simulink model "simscape_robot_delta_v8"  (R2024b)
settings: Solver=ode15s  StartTime=0.0  StopTime=20.0  FixedStep=1e-3  RelTol=1e-3
model workspace (MAT data in the model file):
  kd1 = 14
  kd2 = 13.6
  kd3 = 37.9
  ki1 = 39
  ki2 = 36
  ki3 = 11.6
  kp1 = 12.6
  kp2 = 12.2
  kp3 = 14.4
values from neighbouring files (symbols this model uses):
  N = floor(size(err,1)/window)    [grafica_error.m]
undefined symbols (not defined in the file or in its folder): X, Y, Z
libraries: sm_lib x72, nesl_utility x7
(part 3 of 3)

== matlab function simscape_robot_delta_v8/Inverse Kinematics ==
  data: Pd input; phi_d output
function phi_d = CI(Pd)
%%%%%%%%%%%%%%%%%%%%%%%%%%
    Xp=Pd(1);
    Yp=Pd(2);
    Zp=Pd(3);
    %%%%%%%%%%%%%%%%%%%%%%%%%%
    % constantes
    L1 = 0.17;
    L2 = 0.32513;
    ra = 0.1;
    rb = 0.0501;
    r = ra - rb;
    theta = [0; 2*pi/3; -2*pi/3]; 

    E = 2*L1*(r - Xp*cos(theta) - Yp*sin(theta));
    F = -2*L1*Zp*[1;1;1];
    G = Xp^2 + Yp^2 + Zp^2 + r^2 + L1^2 - L2^2 - 2*r*(Xp*cos(theta) + Yp*sin(theta));
    sqrt_val = E.^2 + F.^2 - G.^2;
    phi_d = 2*atan((-F - sqrt(sqrt_val))./( G - E));
end

== matlab function simscape_robot_delta_v8/Direct Kinematics ==
  data: phi input; P output
function P=CD(phi)
     % Constantes 
    L1 = 0.17;
    L2 = 0.32513;
    ra = 0.1;
    rb = 0.0501;
    r = ra - rb;
    theta = [0; 2*pi/3; -2*pi/3]; 

    % Posiciones de las articulaciones pasivas
    X=(r+L1*cos(phi)).*cos(theta);
    Y=(r+L1*cos(phi)).*sin(theta);
    Z=L1*sin(phi);

    if abs(Z(3)-Z(1))<1e-4 && abs(Z(2)-Z(1))<1e-4
        
        % Definimos matriz del sistema de ecuaciones
        M=[2*(X(3)-X(1)),2*(Y(3)-Y(1));
           2*(X(2)-X(1)),2*(Y(2)-Y(1))];
        b=[X(3)^2+Y(3)^2-(X(1)^2+Y(1)^2);
           X(2)^2+Y(2)^2-(X(1)^2+Y(1)^2)];
        w=M\b;
        Xc=w(1);
        Yc=w(2);
        % Calculamos Z
        Zc=Z(1)+sqrt(L2^2-(Xc-X(1))^2-(Yc-Y(1))^2);
        % Guardamos la solución
        P=[Xc;Yc;Zc];

    elseif abs(X(2)-X(3))<1e-5 && abs(Z(3)-Z(2))<1e-5 && abs(X(3)-X(1))>1e-5 && abs(Z(3)-Z(1))>1e-5

        a=-(Z(3)-Z(1))/(X(3)-X(1)); b=(X(3)^2-X(1)^2+Y(3)^2-Y(1)^2+Z(3)^2-Z(1)^2)/(2*(X(3)-X(1)));
        A=a^2+1; B=2*a*(b-X(3))-2*Z(3); C=(b-X(3))^2+Y(3)^2-L2^2+Z(3)^2;
        Zmas=(-B+sqrt(B^2-4*A*C))/(2*A);
        Xmas=a*Zmas+b;
        Ymas=0;
        P=[Xmas;Ymas;Zmas];
        
    else
        % Definimos coeficientes auxiliares
        a11=2*(X(3)-X(1)); a21=2*(X(3)-X(2));
        a12=2*(Y(3)-Y(1)); a22=2*(Y(3)-Y(2));
        a13=2*(Z(3)-Z(1)); a23=2*(Z(3)-Z(2));

        b1=X(3)^2+Y(3)^2+Z(3)^2-(X(1)^2+Y(1)^2+Z(1)^2);
        b2=X(3)^2+Y(3)^2+Z(3)^2-(X(2)^2+Y(2)^2+Z(2)^2);

        a1=a11/a13-a21/a23; a2=a12/a13-a22/a23; a3=b2/a23-b1/a13;
        a4=-a2/a1; a5=-a3/a1;
        a6=-(a21*a4+a22)/a23; a7=(b2-a21*a5)/a23;

        A=a4^2+1+a6^2;
        B=2*a4*(a5-X(1))-2*Y(1)+2*a6*(a7-Z(1));
        C=a5*(a5-2*X(1))+a7*(a7-2*Z(1))+X(1)^2+Y(1)^2+Z(1)^2-L2^2;

        % Calculamos las dos posibles soluciones
        Ymas=(-B+sqrt(B^2-4*A*C))/(2*A); Xmas=a4*Ymas+a5; Zmas=a6*Ymas+a7;
        Ymenos=(-B-sqrt(B^2-4*A*C))/(2*A); Xmenos=a4*Ymenos+a5; Zmenos=a6*Ymenos+a7;
        
        % Guardamos la solución correcta
        if Zmas>0
            P=[Xmas;Ymas;Zmas]; 
        else
            P=[Xmenos;Ymenos;Zmenos];
        end
    end
end

== matlab function simscape_robot_delta_v8/Trajectory planning ==
  data: t input; Pd output
function Pd = Plan_tray(t)
        %% Descripción
        %% Parámetros
        r=0.15; %0.1
        h=0; %0.3;
        k=0; %0.3;
        %% Ecuaciones
        xd=r*cos(t)+h;
        yd=r*sin(t)+k;
        zd=0.23;
        Pd=[xd; yd; zd];
    end

== matlab function simscape_robot_delta_v8/Dynamics ==
  data: phi input; P input; P_ddot input; tau input; phi_ddot output
function phi_ddot=Dinamica(phi,P,P_ddot,tau)
    % Constantes
    L1 = 0.17;
    L2 = 0.32513;
    ra = 0.1;
    rb = 0.0501;
    r = ra - rb;
    mp=0.2;
    m1=0.103;
    m2=0.124;
    Im=0.01;
    g=9.81;
    Fpx=0;
    Fpy=0;
    Fpz=0;
    theta = [0; 2*pi/3; -2*pi/3];
    G=[0;0;g];
    Fext=[Fpx;Fpy;Fpz];

    % Constantes auxiliares
    Mpos=(mp+3*m2)/2;
    Mphi=m1/2+m2;
    I=Im+m1*L1^2/3+m2*L1^2;
    
    % Posición del efector final
    Xp=P(1);
    Yp=P(2);
    Zp=P(3);
    
    % Posiciones de las articulaciones pasivas
    X=(r+L1*cos(phi)).*cos(theta);
    Y=(r+L1*cos(phi)).*sin(theta);
    Z=L1*sin(phi);

    % Se definen matrices y vectores para el sistema de ecuaciones
    %de las variables de posición 
    A=[Xp-X(1),Xp-X(2),Xp-X(3);
       Yp-Y(1),Yp-Y(2),Yp-Y(3);
       Zp-Z(1),Zp-Z(2),Zp-Z(3)];
    Lambda=A\(Mpos*(P_ddot+G)-0.5*Fext);
    
    % Se definen matrices y vectores para el sistema de ecuaciones
    %de las variables de phi_1i
    B=2*L1*((-r+Xp*cos(theta)+Yp*sin(theta)).*sin(phi)-Zp*cos(phi));
    phi_ddot=(tau-Mphi*g*L1*cos(phi)+B.*Lambda)/I;
end

== matlab function simscape_robot_delta_v8/Aceleration trajectory planning ==
  data: t input; Pd_ddot output
function Pd_ddot = Acel_Plan_tray(t)
        %% Descripción
        %% Parámetros
        r=0.15; %0.1
        %% Ecuaciones
        xd_ddot=-r*cos(t);
        yd_ddot=-r*sin(t);
        zd_ddot=0;
        Pd_ddot=[xd_ddot; yd_ddot; zd_ddot];
    end
